simulink model "PC_drone_Simulation"  (R2014a)
settings: Solver=ode45  StartTime=0  StopTime=20  FixedStep=0.02  MaxStep=0.06  RelTol=1e-3
model workspace (MAT data in the model file):
  Sig = Simulink.Signal
  Sig.DataType = 'auto'
  Sig.Dimensions = -1
  Sig.DimensionsMode = 'auto'
  Sig.Complexity = 'auto'
  Sig.SampleTime = -1
  Sig.SamplingMode = 'auto'
Description:
  | This is a configurable quadcopter simulation.
  | This Simulink model demonstates attitude control.
  | 
  | Additional quadcopter modeling and simulation materials available at:
  | github.com/dch33/Quad-Sim
  | 
  | Copyright (C) 2014 D. Hartman, K. Landis, S. Moreno, J. Kim, M. Mehrer
  | 
  | License:
  |     This program is free software: you can redistribute it and/or modify
  |     it under the terms of the GNU LESSER GENERAL PUBLIC LICENSE as published by
  |     the Free Software Foundation, either version 3 of the License, or
  |     (at your option) any later version.
  | 
  |     This program is distributed in the hope that it will be useful,
  |     but WITHOUT ANY WARRANTY; without even the implied warranty of
  |     MERCHANTABILITY or FITNESS FOR A PARTICULAR PURPOSE.  See the
  |     GNU General Public License for more details.
  | 
  |     You should have received a copy of the GNU LESSER GENERAL PUBLIC LICENSE
  |     along with this program.  If not, see <http://www.gnu.org/licenses/>.
settings Model: ModifiedComment=USER -- Fri Dec 16 02:54:01 2016 -- Version 1.130  Creator=David Hartman  LastModifiedBy=khsun
settings Model: ModifiedHistory=|
  | USER -- Fri Dec 16 02:54:01 2016 -- Version 1.130
  | 
  | 
  | USER -- Fri Dec 16 02:54:01 2016 -- Version 1.130
  | 
  | 
  | USER -- Fri Dec 16 02:34:16 2016 -- Version 1.127
  | 
  | 
  | USER -- Fri Dec 16 02:34:16 2016 -- Version 1.127
  | 
  | 
  | USER -- Fri Dec 16 02:34:16 2016 -- Version 1.127
  | 
  | 
  | USER -- Fri Dec 16 01:26:53 2016 -- Version 1.126
  | 
  | 
  | USER -- Fri Dec 16 01:24:30 2016 -- Version 1.125
  | 
  | 
  | USER -- Fri Dec 16 01:23:22 2016 -- Version 1.124
  | 
  | 
  | USER -- Fri Dec 16 01:18:41 2016 -- Version 1.123
  | 
  | 
  | USER -- Fri Dec 16 01:06:27 2016 -- Version 1.121
  | 
  | 
  | USER -- Fri Dec 16 01:06:27 2016 -- Version 1.121
  | 
  | 
  | USER -- Fri Dec 16 01:06:15 2016 -- Version 1.120
  | 
  | 
  | USER -- Fri Dec 16 01:03:01 2016 -- Version 1.119
  | 
  | 
  | USER -- Fri Dec 16 01:02:34 2016 -- Version 1.118
  | 
  | 
  | USER -- Fri Dec 16 01:00:57 2016 -- Version 1.117
  | 
  | 
  | USER -- Fri Dec 16 00:59:40 2016 -- Version 1.116
  | 
  | 
  | USER -- Fri Dec 16 00:53:32 2016 -- Version 1.114
  | 
  | 
  | USER -- Fri Dec 16 00:53:32 2016 -- Version 1.114
  | 
  | 
  | USER -- Fri Dec 16 00:52:02 2016 -- Version 1.113
  | 
  | 
  | USER -- Fri Dec 16 00:41:04 2016 -- Version 1.112
  | 
  | 
  | USER -- Fri Dec 16 00:30:29 2016 -- Version 1.111
  | 
  | 
  | sstal -- Sun Dec 04 04:26:47 2016 -- Version 1.110
  | 
  | 
  | sstal -- Sun Dec 04 02:45:09 2016 -- Version 1.109
  | 
  | 
  | sstal -- Sun Dec 04 02:38:56 2016 -- Version 1.108
  | 
  | 
  | sstal -- Sun Dec 04 02:33:04 2016 -- Version 1.107
  | 
  | 
  | sstal -- Sun Dec 04 02:24:27 2016 -- Version 1.106
  | 
  | 
  | sstal -- Sun Dec 04 02:10:13 2016 -- Version 1.105
  | 
  | 
  | sstal -- Sun Dec 04 02:09:16 2016 -- Version 1.104
  | 
  | 
  | sstal -- Sun Dec 04 01:58:29 2016 -- Version 1.103
  | 
  | 
  | sstal -- Sun Dec 04 01:49:36 2016 -- Version 1.102
  | 
  | 
  | sstal -- Sat Dec 03 22:54:16 2016 -- Version 1.101
  | 
  | 
  | sstal -- Sat Dec 03 22:52:17 2016 -- Version 1.100
  | 
  | 
  | sstal -- Fri Dec 02 21:35:40 2016 -- Version 1.99
  | 
  | 
  | sstal -- Fri Dec 02 20:50:23 2016 -- Version 1.98
  | 
  | 
  | sstal -- Fri Dec 02 19:45:10 2016 -- Version 1.97
  | 
  | 
  | sstal -- Fri Dec 02 16:57:20 2016 -- Version 1.96
  | 
  | 
  | SKY 05 -- Fri Dec 02 00:32:51 2016 -- Version 1.95
  | 
  | 
  | SKY 05 -- Thu Dec 01 23:20:58 2016 -- Version 1.94
  | 
  | 
  | SKY 05 -- Thu Dec 01 12:57:28 2016 -- Version 1.93
  | 
  | 
  | SKY 05 -- Wed Nov 30 14:36:02 2016 -- Version 1.92
  | 
  | 
  | SKY 03 -- Tue Nov 29 23:04:25 2016 -- Version 1.91
  | 
  | 
  | SKY 03 -- Tue Nov 29 22:01:09 2016 -- Version 1.90
  | 
  | 
  | SKY 03 -- Tue Nov 29 21:15:44 2016 -- Version 1.89
  | 
  | 
  | SKY 03 -- Tue Nov 29 19:16:05 2016 -- Version 1.88
  | 
  | 
  | SKY 03 -- Tue Nov 29 18:05:54 2016 -- Version 1.87
  | 
  | 
  | SKY 03 -- Tue Nov 29 14:57:27 2016 -- Version 1.86
  | 
  | 
  | SKY 03 -- Tue Nov 29 14:50:24 2016 -- Version 1.85
  | 
  | 
  | SKY 03 -- Tue Nov 29 14:29:54 2016 -- Version 1.84
  | 
  | 
  | SKY 03 -- Tue Nov 29 14:29:26 2016 -- Version 1.83
  | 
  | 
  | SKY 03 -- Tue Nov 29 14:12:46 2016 -- Version 1.82
  | 
  | 
  | SKY 05 -- Tue Nov 29 01:43:26 2016 -- Version 1.81
  | 
  | 
  | SKY 05 -- Tue Nov 29 00:54:08 2016 -- Version 1.80
  | 
  | 
  | SKY 05 -- Tue Nov 29 00:24:35 2016 -- Version 1.79
  | 
  | 
  | SKY 05 -- Tue Nov 29 00:14:25 2016 -- Version 1.78
  | 
  | 
  | SKY 05 -- Tue Nov 29 00:11:46 2016 -- Version 1.77
  | 
  | 
  | SKY 05 -- Tue Nov 29 00:10:44 2016 -- Version 1.76
  | 
  | 
  | SKY 05 -- Mon Nov 28 23:29:36 2016 -- Version 1.75
  | 
  | 
  | SKY 05 -- Mon Nov 28 23:29:19 2016 -- Version 1.74
  | 
  | 
  | SKY 05 -- Mon Nov 28 23:23:54 2016 -- Version 1.73
  | 
  | 
  | SKY 05 -- Mon Nov 28 17:23:20 2016 -- Version 1.72
  | 
  | 
  | SKY 05 -- Mon Nov 28 15:05:10 2016 -- Version 1.71
  | 
  | 
  | SKY 05 -- Mon Nov 28 15:03:54 2016 -- Version 1.70
  | 
  | 
  | SKY 05 -- Mon Nov 28 15:01:18 2016 -- Version 1.69
  | 
  | 
  | SKY 05 -- Mon Nov 28 14:59:20 2016 -- Version 1.68
  | 
  | 
  | SKY15 -- Tue Dec 27 23:01:23 2016 -- Version 1.67
  | 
  | 
  | SKY 05 -- Sun Nov 27 00:40:54 2016 -- Version 1.66
  | 
  | 
  | SKY 05 -- Sun Nov 27 00:39:41 2016 -- Version 1.65
  | 
  | 
  | SKY 05 -- Sun Nov 27 00:35:40 2016 -- Version 1.64
  | 
  | 
  | SKY 05 -- Sun Nov 27 00:31:30 2016 -- Version 1.63
  | 
  | 
  | SKY 05 -- Sat Nov 26 23:45:19 2016 -- Version 1.62
  | 
  | 
  | SKY 05 -- Sat Nov 26 22:11:47 2016 -- Version 1.61
  | 
  | 
  | SKY 05 -- Sat Nov 26 22:06:18 2016 -- Version 1.60
  | 
  | 
  | SKY 05 -- Sat Nov 26 21:42:29 2016 -- Version 1.59
  | 
  | 
  | khsun -- Sat Nov 26 20:51:23 2016 -- Version 1.58
  | 
  | 
  | khsun -- Sat Nov 26 20:25:48 2016 -- Version 1.57
  | 
  | 
  | khsun -- Sat Nov 26 20:20:04 2016 -- Version 1.56
  | 
  | 
  | khsun -- Sat Nov 26 20:15:53 2016 -- Version 1.55
  | 
  | 
  | khsun -- Sat Nov 26 19:10:38 2016 -- Version 1.54
  | 
  | 
  | khsun -- Sat Nov 26 18:25:01 2016 -- Version 1.53
  | 
  | 
  | khsun -- Sat Nov 26 17:24:24 2016 -- Version 1.52
  | 
  | 
  | khsun -- Sat Nov 26 17:17:34 2016 -- Version 1.51
  | 
  | 
  | khsun -- Sat Nov 26 16:55:15 2016 -- Version 1.50
  | 
  | 
  | khsun -- Sat Nov 26 16:52:55 2016 -- Version 1.49
  | 
  | 
  | khsun -- Sat Nov 26 16:49:39 2016 -- Version 1.48
  | 
  | 
  | khsun -- Sat Nov 26 16:21:13 2016 -- Version 1.47
  | 
  | 
  | khsun -- Sat Nov 26 16:21:01 2016 -- Version 1.46
  | 
  | 
  | khsun -- Sat Nov 26 16:20:27 2016 -- Version 1.45
  | 
  | 
  | khsun -- Sat Nov 26 12:23:16 2016 -- Version 1.44
  | 
  | 
  | khsun -- Sat Nov 26 12:22:44 2016 -- Version 1.43
  | 
  | 
  | khsun -- Sat Nov 26 12:09:40 2016 -- Version 1.42
  | 
  | 
  | khsun -- Fri Nov 25 12:53:36 2016 -- Version 1.41
  | 
  | 
  | khsun -- Thu Nov 24 15:51:55 2016 -- Version 1.40
  | 
  | 
  | khsun -- Thu Nov 24 15:40:52 2016 -- Version 1.39
  | 
  | 
  | khsun -- Thu Nov 24 15:25:38 2016 -- Version 1.38
  | 
  | 
  | khsun -- Thu Nov 24 15:20:43 2016 -- Version 1.37
  | 
  | 
  | khsun -- Thu Nov 24 15:15:05 2016 -- Version 1.36
  | 
  | 
  | khsun -- Thu Nov 24 15:14:02 2016 -- Version 1.35
  | 
  | 
  | khsun -- Thu Nov 24 11:17:00 2016 -- Version 1.34
  | 
  | 
  | khsun -- Wed Nov 23 23:17:43 2016 -- Version 1.33
  | 
  | 
  | khsun -- Wed Nov 23 17:41:56 2016 -- Version 1.31
  | 
  | 
  | khsun -- Wed Nov 23 17:41:56 2016 -- Version 1.31
  | 
  | 
  | khsun -- Tue Nov 22 22:20:06 2016 -- Version 1.30
  | 
  | 
  | khsun -- Tue Nov 22 22:09:32 2016 -- Version 1.29
  | 
  | 
  | khsun -- Tue Nov 22 22:08:32 2016 -- Version 1.28
  | 
  | 
  | khsun -- Tue Nov 22 22:07:24 2016 -- Version 1.27
  | 
  | 
  | khsun -- Tue Nov 22 22:06:29 2016 -- Version 1.26
  | 
  | 
  | khsun -- Tue Nov 22 22:06:06 2016 -- Version 1.25
  | 
  | 
  | khsun -- Tue Nov 22 22:03:53 2016 -- Version 1.24
  | 
  | 
  | khsun -- Tue Nov 22 21:01:42 2016 -- Version 1.23
  | 
  | 
  | khsun -- Tue Nov 22 20:59:39 2016 -- Version 1.22
  | 
  | 
  | khsun -- Tue Nov 22 20:24:50 2016 -- Version 1.21
  | 
  | 
  | khsun -- Tue Nov 22 20:14:42 2016 -- Version 1.20
  | 
  | 
  | khsun -- Tue Nov 22 16:24:10 2016 -- Version 1.19
  | 
  | 
  | khsun -- Tue Nov 22 16:10:18 2016 -- Version 1.18
  | 
  | 
  | khsun -- Tue Nov 22 11:35:43 2016 -- Version 1.17
  | 
  | 
  | khsun -- Tue Nov 22 10:54:15 2016 -- Version 1.16
  | 
  | 
  | khsun -- Mon Nov 21 21:57:53 2016 -- Version 1.15
  | 
  | 
  | khsun -- Mon Nov 21 21:12:45 2016 -- Version 1.14
  | 
  | 
  | khsun -- Sun Nov 20 22:34:28 2016 -- Version 1.13
  | 
  | 
  | khsun -- Sun Nov 20 19:39:17 2016 -- Version 1.12
  | 
  | 
  | khsun -- Sun Nov 20 17:26:15 2016 -- Version 1.11
  | 
  | 
  | khsun -- Sun Nov 20 17:01:09 2016 -- Version 1.10
  | 
  | 
  | khsun -- Sun Nov 20 15:27:38 2016 -- Version 1.9
  | 
  | 
  | khsun -- Sun Nov 20 15:24:18 2016 -- Version 1.8
  | 
  | 
  | khsun -- Sun Nov 20 15:24:12 2016 -- Version 1.7
  | 
  | 
  | khsun -- Sun Nov 20 14:36:24 2016 -- Version 1.6
  | 
  | 
  | davidhartman -- Fri Jun 06 23:19:51 2014 -- Version 1.5
  | 
  | 
  | davidhartman -- Fri Jun 06 22:53:10 2014 -- Version 1.3
settings SolverCC: AutoInsertRateTranBlk=on
settings DataIOCC: LimitDataPoints=off  SignalLogging=off
settings OptimizationCC: InlineParams=on
settings DebuggingCC: UnderspecifiedInitializationDetection=Classic  UniqueDataStoreMsg=warning  StateNameClashWarn=warning  StrictBusMsg=WarnOnBusTreatedAsVector

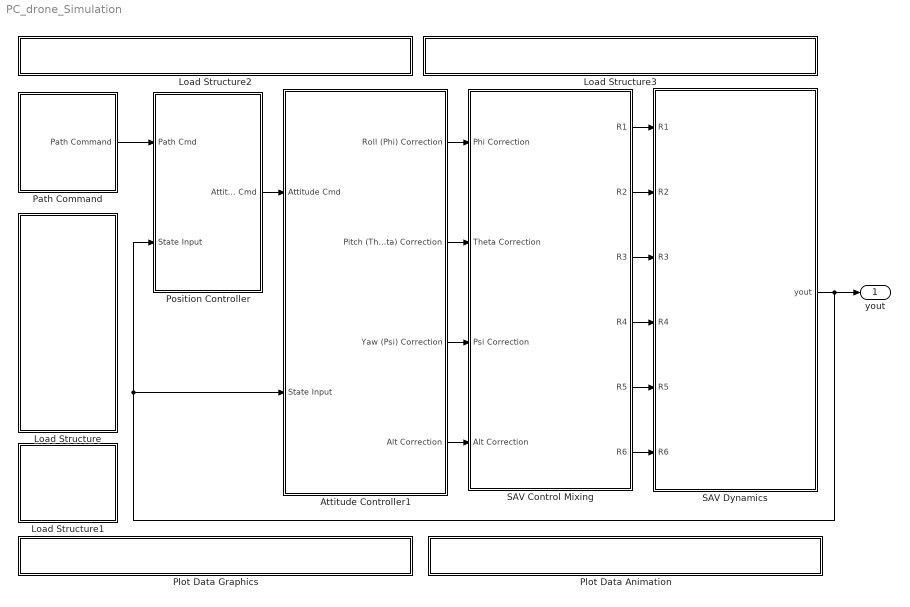
== system PC_drone_Simulation ==
  Attitude Controller1 : Subsystem
  Load Structure : Subsystem
      settings: OpenFcn=|
      | uiopen('load')
      | if ((exist('IC')==1) && (exist('quadModel')==1) && (exist('path')==1))
      | set_param(bdroot, 'SimulationCommand', 'update')
      | end
      mask Display: fprintf('LOAD:\nTimeseries\nPath\nCommands,\ndrone\nModel, Or\nInitial\nConditions');
  Load Structure1 : Subsystem
      settings: OpenFcn=|
      | if (exist('IC')==1 && exist('quadModel')==1 && exist('yout') && exist('tout'))
      | saveSimResults()
      | else
      | msgbox('No Data To Save!')
      | end
      mask Display: fprintf('SAVE:\nSimulation\nResults');
  Load Structure2 : Subsystem
      settings: OpenFcn=|
      | if exist('GUI_Modeling') == 2,
      | run('GUI_Modeling')
      | 
      | else
      | 
      | msgbox('The desired GUI must be first added to MATLABs path.')
      | 
      | end
      mask Display: fprintf('OPEN GUI: Build New \n Model');
  Load Structure3 : Subsystem
      settings: OpenFcn=|
      | if exist('GUI_IC') == 2,
      | run('GUI_IC')
      | 
      | else
      | 
      | msgbox('The desired GUI must be first added to MATLABs path.')
      | 
      | end
      mask Display: fprintf('OPEN GUI: Create Initial \n Conditions');
  Path Command : Subsystem  mask{Interpolate=on, OutputAfterFinalValue=Holding final value}
      mask prompts: Interpolate "Interpolate X, Y, Z, and Psi command data?"; OutputAfterFinalValue "Form output after final data value by:"
      mask help:
      | Selecting the Interpolate data checkbox causes position commands to be
      | linearly interpolated. For additional options related to the Timeseries
      | "path" commands, look under the block and click on the Timeseries From
      | Workspace blocks.
      mask TypeOptions Interpolate: X Timeseries From Wkspace/Interpolate | Y Timeseries From Wkspace/Interpolate | Z Timeseries From Wkspace/Interpolate | Psi Timeseries From Wkspace/Interpolate
      mask TypeOptions OutputAfterFinalValue: X Timeseries From Wkspace/OutputAfterFinalValue | Y Timeseries From Wkspace/OutputAfterFinalValue | Z Timeseries From Wkspace/OutputAfterFinalValue | Psi Timeseries From Wkspace/OutputAfterFinalValue
  Plot Data Animation : Subsystem
      settings: OpenFcn=|
      | if exist('droneAnim4') == 2,
      |     if exist('yout')
      | 	run('droneAnim4');
      |     else
      |     msgbox('Simulation must be run before data can be plotted.');
      |     end
      | else                                                                          msgbox('The desired GUI must be first added to MATLABs path.')
      | end
      mask Display: fprintf('OPEN GUI: Flight Animation')
  Plot Data Graphics : Subsystem
      settings: OpenFcn=|
      | if exist('yout')
      | yout = evalin('base', 'yout');
      | tout = evalin('base', 'tout');
      | dronePlots(yout, tout)
      | else
      | msgbox('Simulation must be run before data can be plotted.')
      | end
      mask Display: fprintf('OPEN PLOT: State Data')
  Position Controller : Subsystem
  SAV Control Mixing : Subsystem
  SAV Dynamics : Subsystem
  yout : Outport
  wires:
  Position Controller/1(Attitude Cmd) -> Attitude Controller1/1(Attitude Cmd)
  Path Command/1("Path Command ") -> Position Controller/1(Path Cmd)
  Attitude Controller1/1(Roll (Phi) Correction) -> SAV Control Mixing/1(Phi Correction)
  Attitude Controller1/2(Pitch (Theta) Correction) -> SAV Control Mixing/2(Theta Correction)
  Attitude Controller1/3(Yaw (Psi) Correction) -> SAV Control Mixing/3(Psi Correction)
  Attitude Controller1/4(Alt Correction) -> SAV Control Mixing/4(Alt Correction)
  SAV Control Mixing/1(R1) -> SAV Dynamics/1(R1)
  SAV Control Mixing/2(R2) -> SAV Dynamics/2(R2)
  SAV Control Mixing/3(R3) -> SAV Dynamics/3(R3)
  SAV Control Mixing/4(R4) -> SAV Dynamics/4(R4)
  SAV Control Mixing/5(R5) -> SAV Dynamics/5(R5)
  SAV Control Mixing/6(R6) -> SAV Dynamics/6(R6)
  SAV Dynamics/1(yout) -> Attitude Controller1/2(State Input), Position Controller/2(State Input), yout/1

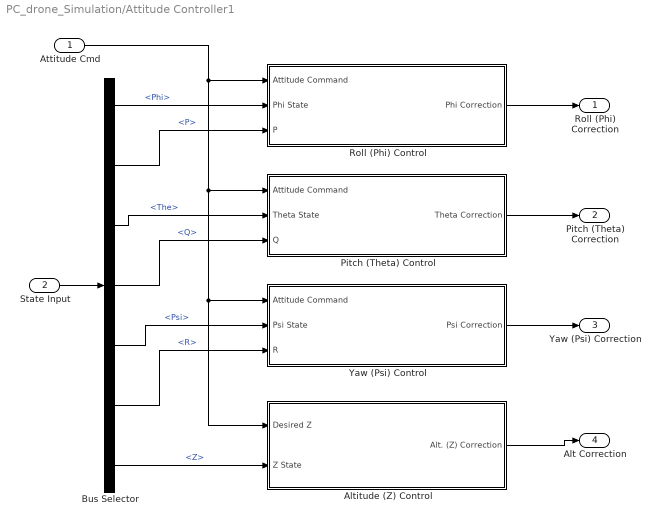
== system PC_drone_Simulation/Attitude Controller1 ==
  Attitude Cmd : Inport
  State Input : Inport  Port=2
  Altitude (Z) Control : Subsystem  mask{Kpz=10, Kiz=0, Kdz=3, LimitOutput=off, USat=1, LSat=-1, GOffset=0}
      mask prompts: Kpz "Kp"; Kiz "Ki"; Kdz "Kd"; LimitOutput "Integral Saturation?"; USat "Upper saturation limit:"; LSat "Lower saturation limit:"; GOffset "Gravity Feedforward"
      mask help:
      | Adjust PID controller gains through this mask interface, or "look under mask" for more detailed adjustments.
      |
      | Note: Gravity Offset will not appear on block face as a value until simulation is run if it is the result of a formula involving the quadcopter model parameters.
      mask TypeOptions Kpz: Kpz/Gain
      mask TypeOptions Kiz: Kiz/Gain
      mask TypeOptions Kdz: Kdz/Gain
      mask TypeOptions LimitOutput:
      | Integrator
      | Limited/LimitOutput
      mask TypeOptions USat:
      | Integrator
      | Limited/UpperSaturationLimit
      mask TypeOptions LSat:
      | Integrator
      | Limited/LowerSaturationLimit
      mask TypeOptions GOffset: Gravity Offset (Level Flight)/Value
      mask Display:
      | fprintf(['Kp = ' num2str(Kpz) '\n' ...
      |     'Ki = ' num2str(Kiz) '\n' ...
      |     'Kd = ' num2str(Kdz) '\n' ...
      |     'Integral Saturation: ' LimitOutput]);
      | if strcmp(LimitOutput,'on')
      |     fprintf([' \n' ' \n' ' \n' ' \n' ' \n' '\n' ...
      |         'Limits: ' num2str(USat) ' to ' num2str(LSat)]);
      | end
  Bus Selector : BusSelector  OutputSignals=Phi,P,The,Q,Psi,R,Z
  Pitch (Theta) Control : Subsystem  mask{Kpt=5, Kit=1, Kdt=3, LimitOutput=off, USat=1, LSat=-1}
      mask prompts: Kpt "Kp"; Kit "Ki"; Kdt "Kd"; LimitOutput "Integral Saturation?"; USat "Upper saturation limit:"; LSat "Lower saturation limit:"
      mask help: Adjust PID controller gains through this mask interface, or "look under mask" for more detailed adjustments.
      mask TypeOptions Kpt: Kpt/Gain
      mask TypeOptions Kit: Kit/Gain
      mask TypeOptions Kdt: Kdt/Gain
      mask TypeOptions LimitOutput:
      | Integrator
      | Limited/LimitOutput
      mask TypeOptions USat:
      | Integrator
      | Limited/UpperSaturationLimit
      mask TypeOptions LSat:
      | Integrator
      | Limited/LowerSaturationLimit
      mask Display:
      | fprintf(['Kp = ' num2str(Kpt) '\n' ...
      |     'Ki = ' num2str(Kit) '\n' ...
      |     'Kd = ' num2str(Kdt) '\n' ...
      |     'Integral Saturation: ' LimitOutput]);
      | if strcmp(LimitOutput,'on')
      |     fprintf([' \n' ' \n' ' \n' ' \n' '\n' ...
      |         'Limits: ' num2str(USat) ' to ' num2str(LSat)]);
      | end
  "Roll (Phi) Control " : Subsystem  mask{Kpp=5, Kip=1, Kdp=3, LimitOutput=off, USat=1, LSat=-1}
      mask prompts: Kpp "Kp"; Kip "Ki"; Kdp "Kd"; LimitOutput "Integral Saturation:"; USat "Upper saturation limit:"; LSat "Lower saturation limit:"
      mask help:
      | Adjust PID controller gains through this mask interface, or "look under mask"
      | for more detailed adjustments.
      mask TypeOptions Kpp: Kpp/Gain
      mask TypeOptions Kip: Kip/Gain
      mask TypeOptions Kdp: Kdp/Gain
      mask TypeOptions LimitOutput:
      | Integrator
      | Limited/LimitOutput
      mask TypeOptions USat:
      | Integrator
      | Limited/UpperSaturationLimit
      mask TypeOptions LSat:
      | Integrator
      | Limited/LowerSaturationLimit
      mask Display:
      | fprintf(['Kp = ' num2str(Kpp) '\n' ...
      |     'Ki = ' num2str(Kip) '\n' ...
      |     'Kd = ' num2str(Kdp) '\n'...
      |     'Integral Saturation: ' LimitOutput]);
      | if strcmp(LimitOutput,'on')
      |     fprintf([' \n' ' \n' ' \n' ' \n' '\n' ...
      |         'Limits: ' num2str(USat) ' to ' num2str(LSat)]);
      | end
  Yaw (Psi) Control : Subsystem  mask{Kps=4, Kis=1, Kds=2, LimitOutput=off, USat=1, LSat=-1}
      mask prompts: Kps "Kp"; Kis "Ki"; Kds "Kd"; LimitOutput "Integral Saturation?"; USat "Upper saturation limit:"; LSat "Lower saturation limit:"
      mask help: Adjust PID controller gains through this mask interface, or "look under mask" for more detailed adjustments.
      mask TypeOptions Kps: Kps/Gain
      mask TypeOptions Kis: Kit/Gain
      mask TypeOptions Kds: Kds/Gain
      mask TypeOptions LimitOutput:
      | Integrator
      | Limited/LimitOutput
      mask TypeOptions USat:
      | Integrator
      | Limited/UpperSaturationLimit
      mask TypeOptions LSat:
      | Integrator
      | Limited/LowerSaturationLimit
      mask Display:
      | fprintf(['Kp = ' num2str(Kps) '\n' ...
      |     'Ki = ' num2str(Kis) '\n' ...
      |     'Kd = ' num2str(Kds) '\n' ...
      |     'Integral Saturation: ' LimitOutput]);
      | if strcmp(LimitOutput,'on')
      |     fprintf([' \n' ' \n' ' \n' ' \n' '\n' ...
      |         'Limits: ' num2str(USat) ' to ' num2str(LSat)]);
      | end
  Roll (Phi) Correction : Outport
  Pitch (Theta) Correction : Outport  Port=2
  Yaw (Psi) Correction : Outport  Port=3
  Alt Correction : Outport  Port=4
  wires:
  Bus Selector/3 -> Pitch (Theta) Control/2(Theta State)  "<The>"
  Attitude Cmd/1 -> Altitude (Z) Control/1(Desired Z), Yaw (Psi) Control/1(Attitude Command), Pitch (Theta) Control/1(Attitude Command), "Roll (Phi) Control "/1("Attitude Command ")
  Bus Selector/5 -> Yaw (Psi) Control/2(Psi State)  "<Psi>"
  Yaw (Psi) Control/1(Psi Correction) -> Yaw (Psi) Correction/1
  Pitch (Theta) Control/1(Theta Correction) -> Pitch (Theta) Correction/1
  State Input/1 -> Bus Selector/1
  Bus Selector/1 -> "Roll (Phi) Control "/2(Phi State)  "<Phi>"
  "Roll (Phi) Control "/1(Phi Correction) -> Roll (Phi) Correction/1
  Bus Selector/7 -> Altitude (Z) Control/2(Z State)  "<Z>"
  Altitude (Z) Control/1(Alt. (Z) Correction) -> Alt Correction/1
  Bus Selector/2 -> "Roll (Phi) Control "/3(P)  "<P>"
  Bus Selector/4 -> Pitch (Theta) Control/3(Q)  "<Q>"
  Bus Selector/6 -> Yaw (Psi) Control/3(R)  "<R>"

== system PC_drone_Simulation/Load Structure ==

== system PC_drone_Simulation/Load Structure1 ==

== system PC_drone_Simulation/Load Structure2 ==

== system PC_drone_Simulation/Load Structure3 ==

== system PC_drone_Simulation/Path Command ==
  Bus Creator : BusCreator  Inputs=3
  Bus Selector : BusSelector  OutputSignals=X_cmd,Y_cmd  OutputAsBus=on
  X Timeseries From Wkspace : FromWorkspace  VariableName=path.x  SampleTime=0  OutputAfterFinalValue=Holding final value
  Y Timeseries From Wkspace : FromWorkspace  VariableName=path.y  SampleTime=0  OutputAfterFinalValue=Holding final value
  Z Timeseries From Wkspace : FromWorkspace  VariableName=path.z  SampleTime=0  OutputAfterFinalValue=Holding final value
  "Path Command " : Outport
  tag scope: C=global
  wires:
  X Timeseries From Wkspace/1 -> Bus Creator/1  "X_cmd"
  Y Timeseries From Wkspace/1 -> Bus Creator/2  "Y_cmd"
  Z Timeseries From Wkspace/1 -> Bus Creator/3  "Alt_Cmd"
  Bus Creator/1 -> "Path Command "/1, Bus Selector/1  "Path_Cmd"
  Bus Selector/1 -> [C]  "XY_Cmd"

== system PC_drone_Simulation/Plot Data Animation ==

== system PC_drone_Simulation/Plot Data Graphics ==

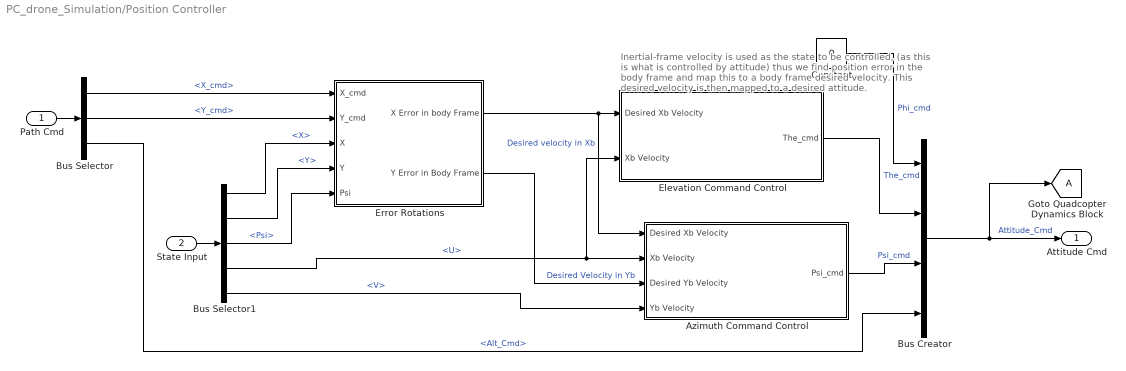
== system PC_drone_Simulation/Position Controller ==
  note: Inertial-frame velocity is used as the state to be controlled,
      | (as this is what is controlled by attitude)
      | thus we find position error in the body frame
      | and map this to a body frame desired velocity. This desired
      | velocity is then mapped to a desired attitude.
  Path Cmd : Inport
  State Input : Inport  Port=2
  Azimuth Command Control : Subsystem  mask{Kp=0.3, Kd=0}
      mask prompts: Kp "Proportional Gain"; Kd "Derivative Gain"
      mask TypeOptions Kp: Kpp/Gain
      mask TypeOptions Kd: Kdp/Gain
      mask Display:
      | fprintf(['Kp = ' num2str(Kp) '\n' ...
      |     'Kd = ' num2str(Kd) '\n']);
  Bus Creator : BusCreator  Inputs='Phi_cmd','The_cmd','Psi_cmd','Alt_Cmd'
  Bus Selector : BusSelector  OutputSignals=X_cmd,Y_cmd,Alt_Cmd
  Bus Selector1 : BusSelector  OutputSignals=X,Y,Psi,U,V
  Constant : Constant  Value=0
  Elevation Command Control : Subsystem  mask{Kp=0.3, Kd=0, ASat=30*pi/180}
      mask prompts: Kp "Proportional Gain:"; Kd "Derivative Gain"; ASat "Attitude Limit (+/- radians):"
      mask TypeOptions Kp: Kpt/Gain
      mask TypeOptions Kd: Kdt/Gain
      mask TypeOptions ASat: Attitude Limits_Theta/UpperLimit
      mask Display:
      | fprintf(['Kp = ' num2str(Kp) '\n' ...
      |     'Kd = ' num2str(Kd) '\n' ...
      |     'Attitude Limit (+/-): ' num2str(ASat*180/pi) '°']);
  Error Rotations : Subsystem
  Attitude Cmd : Outport
  tag scope: A=global
  wires:
  State Input/1 -> Bus Selector1/1
  Path Cmd/1 -> Bus Selector/1
  Bus Creator/1 -> [A], Attitude Cmd/1  "Attitude_Cmd"
  Bus Selector/1 -> Error Rotations/1(X_cmd)  "<X_cmd>"
  Bus Selector/2 -> Error Rotations/2(Y_cmd)  "<Y_cmd>"
  Bus Selector1/1 -> Error Rotations/3(X)  "<X>"
  Bus Selector1/2 -> Error Rotations/4(Y)  "<Y>"
  Bus Selector1/3 -> Error Rotations/5(Psi)  "<Psi>"
  Constant/1 -> Bus Creator/1  "Phi_cmd"
  Elevation Command Control/1(The_cmd) -> Bus Creator/2  "The_cmd"
  Error Rotations/1(X Error in body Frame) -> Azimuth Command Control/1(Desired Xb Velocity), Elevation Command Control/1(Desired Xb Velocity)  "Desired velocity in Xb"
  Error Rotations/2(Y Error in Body Frame) -> Azimuth Command Control/3(Desired Yb Velocity)  "Desired Velocity in Yb"
  Bus Selector1/4 -> Elevation Command Control/2(Xb Velocity), Azimuth Command Control/2(Xb Velocity)  "<U>"
  Bus Selector1/5 -> Azimuth Command Control/4(Yb Velocity)  "<V>"
  Bus Selector/3 -> Bus Creator/4  "<Alt_Cmd>"
  Azimuth Command Control/1(Psi_cmd) -> Bus Creator/3  "Psi_cmd"

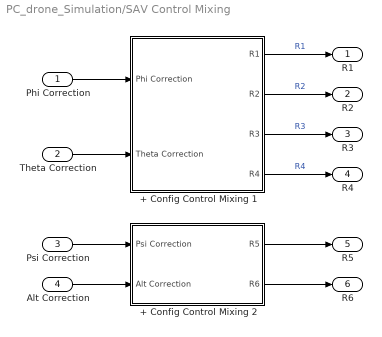
== system PC_drone_Simulation/SAV Control Mixing ==
  Phi Correction : Inport
  Theta Correction : Inport  Port=2
  Psi Correction : Inport  Port=3
  Alt Correction : Inport  Port=4
  + Config Control Mixing 1 : Subsystem
  + Config Control Mixing 2 : Subsystem
  R1 : Outport
  R2 : Outport  Port=2
  R3 : Outport  Port=3
  R4 : Outport  Port=4
  R5 : Outport  Port=5
  R6 : Outport  Port=6
  wires:
  + Config Control Mixing 1/4(R4) -> R4/1  "R4"
  + Config Control Mixing 1/3(R3) -> R3/1  "R3"
  + Config Control Mixing 1/2(R2) -> R2/1  "R2"
  + Config Control Mixing 1/1(R1) -> R1/1  "R1"
  Theta Correction/1 -> + Config Control Mixing 1/2(Theta Correction)
  Phi Correction/1 -> + Config Control Mixing 1/1(Phi Correction)
  Psi Correction/1 -> + Config Control Mixing 2/1(Psi Correction)
  Alt Correction/1 -> + Config Control Mixing 2/2(Alt Correction)
  + Config Control Mixing 2/1(R5) -> R5/1
  + Config Control Mixing 2/2(R6) -> R6/1

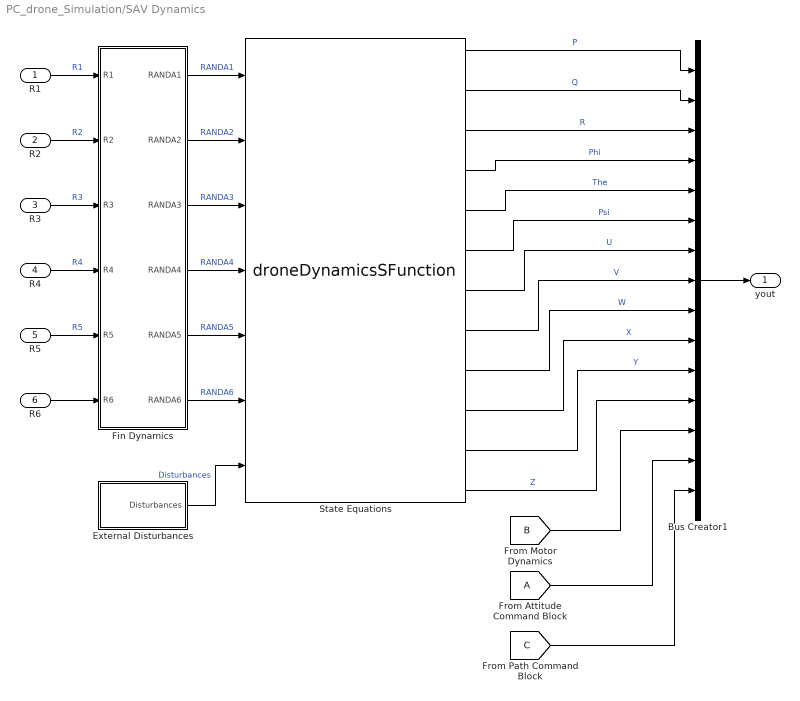
== system PC_drone_Simulation/SAV Dynamics ==
  R1 : Inport
  R2 : Inport  Port=2
  R3 : Inport  Port=3
  R4 : Inport  Port=4
  R5 : Inport  Port=5
  R6 : Inport  Port=6
  Bus Creator1 : BusCreator  Inputs='P','Q','R','Phi','The','Psi','U','V','W','X','Y','Z','mc and RPM','Attitude_Cmd','XY_Cmd'
  External Disturbances : Subsystem
  Fin Dynamics : Subsystem  mask{AOA=50*pi/180}
      mask prompts: AOA "Simulink:blkprm_prompts:SaturateUpLim"
      mask TypeOptions AOA: Signal_Saturation_1/UpperLimit | Signal_Saturation_2/UpperLimit | Signal_Saturation_3/UpperLimit | Signal_Saturation_4/UpperLimit
      mask Display: fprintf(['AOA = ' num2str(AOA*180/pi) '°']);
  State Equations : M-S-Function  FunctionName=droneDynamicsSFunction  Parameters=droneModel, IC
      mask Display:
      | port_label('input', 1, 'RANDA1')
      | port_label('input', 2, 'RANDA2')
      | port_label('input', 3, 'RANDA3')
      | port_label('input', 4, 'RANDA4')
      | port_label('input', 5, 'RANDA5')
      | port_label('input', 6, 'RANDA6')
      | port_label('input', 7, 'Disturbances')
      | port_label('output', 1, 'P')
      | port_label('output', 2, 'Q')
      | port_label('output', 3, 'R')
      | port_label('output', 4, 'Phi')
      | port_label('output', 5, 'The')
      | port_label('output', 6, 'Psi')
      | port_label('output', 7, 'U')
      | port_label('output', 8, 'V')
      | port_label('output', 9, 'W')
      | port_label('output', 10, 'X')
      | port_label('output', 11, 'Y')
      | port_label('output', 12, 'Z')
  yout : Outport
  wires:
  [B] -> Bus Creator1/13
  [A] -> Bus Creator1/14
  R2/1 -> Fin Dynamics/2(R2)  "R2"
  R3/1 -> Fin Dynamics/3(R3)  "R3"
  R4/1 -> Fin Dynamics/4(R4)  "R4"
  R1/1 -> Fin Dynamics/1(R1)  "R1"
  Fin Dynamics/4(RANDA4) -> State Equations/4  "RANDA4"
  Fin Dynamics/3(RANDA3) -> State Equations/3  "RANDA3"
  Fin Dynamics/2(RANDA2) -> State Equations/2  "RANDA2"
  Fin Dynamics/1(RANDA1) -> State Equations/1  "RANDA1"
  State Equations/6 -> Bus Creator1/6  "Psi"
  State Equations/5 -> Bus Creator1/5  "The"
  State Equations/4 -> Bus Creator1/4  "Phi"
  State Equations/3 -> Bus Creator1/3  "R"
  State Equations/2 -> Bus Creator1/2  "Q"
  State Equations/1 -> Bus Creator1/1  "P"
  Bus Creator1/1 -> yout/1
  State Equations/12 -> Bus Creator1/12  "Z"
  State Equations/11 -> Bus Creator1/11  "Y"
  State Equations/10 -> Bus Creator1/10  "X"
  State Equations/9 -> Bus Creator1/9  "W"
  State Equations/7 -> Bus Creator1/7  "U"
  State Equations/8 -> Bus Creator1/8  "V"
  R5/1 -> Fin Dynamics/5(R5)  "R5"
  R6/1 -> Fin Dynamics/6(R6)
  Fin Dynamics/5(RANDA5) -> State Equations/5  "RANDA5"
  Fin Dynamics/6(RANDA6) -> State Equations/6  "RANDA6"
  External Disturbances/1("Disturbances ") -> State Equations/7  "Disturbances"
  [C] -> Bus Creator1/15

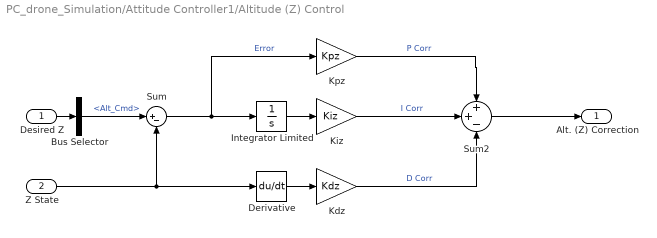
== system PC_drone_Simulation/Attitude Controller1/Altitude (Z) Control ==
  Desired Z : Inport
  Z State : Inport  Port=2
  Bus Selector : BusSelector  OutputSignals=Alt_Cmd
  Derivative : Derivative
  Integrator Limited : Integrator  UpperSaturationLimit=USat  LowerSaturationLimit=LSat
  Kdz : Gain  Gain=Kdz
  Kiz : Gain  Gain=Kiz
  Kpz : Gain  Gain=Kpz
  Sum : Sum  Inputs=|+-
  Sum2 : Sum  Inputs=++-
  Alt. (Z) Correction : Outport
  wires:
  Derivative/1 -> Kdz/1
  Bus Selector/1 -> Sum/1  "<Alt_Cmd>"
  Integrator Limited/1 -> Kiz/1
  Kdz/1 -> Sum2/3  "D Corr"
  Kpz/1 -> Sum2/1  "P Corr"
  Z State/1 -> Sum/2, Derivative/1
  Desired Z/1 -> Bus Selector/1
  Kiz/1 -> Sum2/2  "I Corr"
  Sum/1 -> Integrator Limited/1, Kpz/1  "Error"
  Sum2/1 -> Alt. (Z) Correction/1

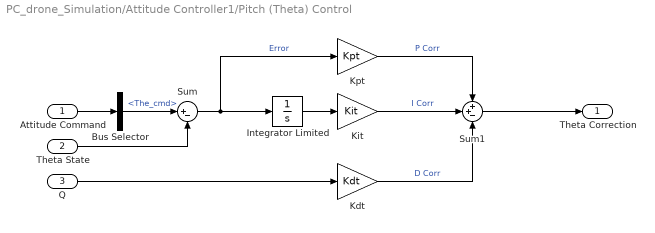
== system PC_drone_Simulation/Attitude Controller1/Pitch (Theta) Control ==
  Attitude Command : Inport
  Theta State : Inport  Port=2
  Q : Inport  Port=3
  Bus Selector : BusSelector  OutputSignals=The_cmd
  Integrator Limited : Integrator  UpperSaturationLimit=USat  LowerSaturationLimit=LSat
  Kdt : Gain  Gain=Kdt
  Kit : Gain  Gain=Kit
  Kpt : Gain  Gain=Kpt
  Sum : Sum  Inputs=|+-
  Sum1 : Sum  Inputs=++-
  Theta Correction : Outport
  wires:
  Bus Selector/1 -> Sum/1  "<The_cmd>"
  Integrator Limited/1 -> Kit/1
  Kit/1 -> Sum1/2  "I Corr"
  Kdt/1 -> Sum1/3  "D Corr"
  Kpt/1 -> Sum1/1  "P Corr"
  Sum1/1 -> Theta Correction/1
  Attitude Command/1 -> Bus Selector/1
  Sum/1 -> Kpt/1, Integrator Limited/1  "Error"
  Theta State/1 -> Sum/2
  Q/1 -> Kdt/1

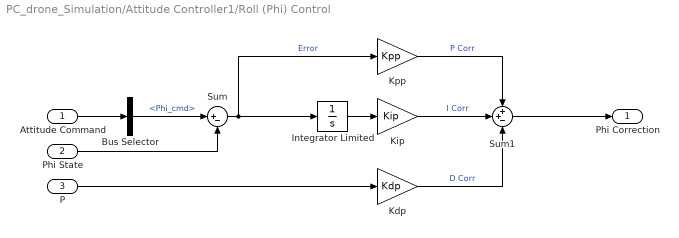
== system PC_drone_Simulation/Attitude Controller1/Roll (Phi) Control  ==
  "Attitude Command " : Inport
  Phi State : Inport  Port=2
  P : Inport  Port=3
  Bus Selector : BusSelector  OutputSignals=Phi_cmd
  Integrator Limited : Integrator  UpperSaturationLimit=USat  LowerSaturationLimit=LSat
  Kdp : Gain  Gain=Kdp
  Kip : Gain  Gain=Kip
  Kpp : Gain  Gain=Kpp
  Sum : Sum  Inputs=|+-
  Sum1 : Sum  Inputs=++-
  Phi Correction : Outport
  wires:
  Bus Selector/1 -> Sum/1  "<Phi_cmd>"
  "Attitude Command "/1 -> Bus Selector/1
  Integrator Limited/1 -> Kip/1
  Kip/1 -> Sum1/2  "I Corr"
  Kdp/1 -> Sum1/3  "D Corr"
  Kpp/1 -> Sum1/1  "P Corr"
  Sum1/1 -> Phi Correction/1
  Sum/1 -> Kpp/1, Integrator Limited/1  "Error"
  Phi State/1 -> Sum/2
  P/1 -> Kdp/1

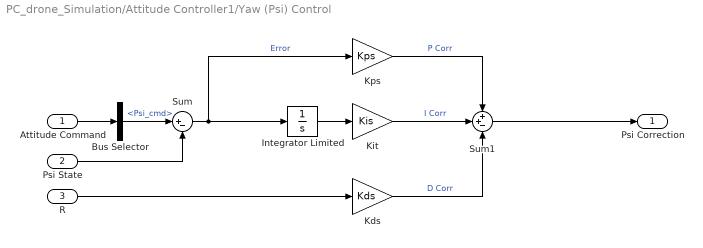
== system PC_drone_Simulation/Attitude Controller1/Yaw (Psi) Control ==
  Attitude Command : Inport
  Psi State : Inport  Port=2
  R : Inport  Port=3
  Bus Selector : BusSelector  OutputSignals=Psi_cmd
  Integrator Limited : Integrator  UpperSaturationLimit=USat  LowerSaturationLimit=LSat
  Kds : Gain  Gain=Kds
  Kit : Gain  Gain=Kis
  Kps : Gain  Gain=Kps
  Sum : Sum  Inputs=|+-
  Sum1 : Sum  Inputs=++-
  Psi Correction : Outport
  wires:
  Bus Selector/1 -> Sum/1  "<Psi_cmd>"
  Integrator Limited/1 -> Kit/1
  Kit/1 -> Sum1/2  "I Corr"
  Kds/1 -> Sum1/3  "D Corr"
  Kps/1 -> Sum1/1  "P Corr"
  Sum1/1 -> Psi Correction/1
  Attitude Command/1 -> Bus Selector/1
  Sum/1 -> Kps/1, Integrator Limited/1  "Error"
  R/1 -> Kds/1
  Psi State/1 -> Sum/2

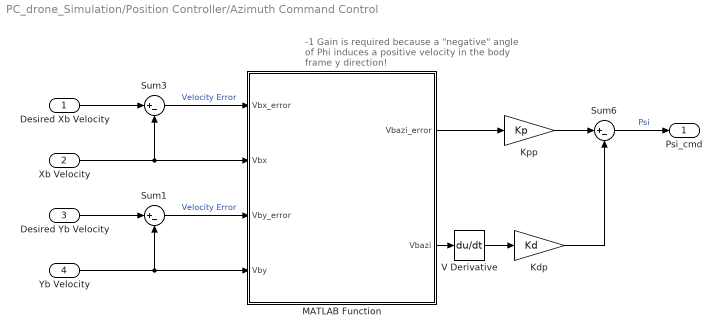
== system PC_drone_Simulation/Position Controller/Azimuth Command Control ==
  note: -1 Gain is required because a "negative"
      | angle of Phi induces a positive velocity
      | in the body frame y direction!
  Desired Xb Velocity : Inport
  Xb Velocity : Inport  Port=2
  Desired Yb Velocity : Inport  Port=3
  Yb Velocity : Inport  Port=4
  Kdp : Gain  Gain=Kd
  Kpp : Gain  Gain=Kp
  MATLAB Function : MATLAB Function  TreatAsAtomicUnit=on
  Sum1 : Sum  Inputs=|+-
  Sum3 : Sum  Inputs=|+-
  Sum6 : Sum  Inputs=|+-
  V Derivative : Derivative
  Psi_cmd : Outport
  wires:
  V Derivative/1 -> Kdp/1
  Kpp/1 -> Sum6/1
  Xb Velocity/1 -> Sum3/2, MATLAB Function/2(Vbx)
  Desired Xb Velocity/1 -> Sum3/1
  Kdp/1 -> Sum6/2
  Yb Velocity/1 -> Sum1/2, MATLAB Function/4(Vby)
  Desired Yb Velocity/1 -> Sum1/1
  Sum3/1 -> MATLAB Function/1(Vbx_error)  "Velocity Error"
  Sum1/1 -> MATLAB Function/3(Vby_error)  "Velocity Error"
  MATLAB Function/1(Vbazi_error) -> Kpp/1
  MATLAB Function/2(Vbazi) -> V Derivative/1
  Sum6/1 -> Psi_cmd/1  "Psi"

== system PC_drone_Simulation/Position Controller/Elevation Command Control ==
  Desired Xb Velocity : Inport
  Xb Velocity : Inport  Port=2
  Attitude Limits_Theta : Saturate  UpperLimit=ASat  LowerLimit=-ASat
  Kdt : Gain  Gain=Kd
  Kpt : Gain  Gain=Kp
  Sum3 : Sum  Inputs=|+-
  Sum6 : Sum  Inputs=|+-
  U Derivative : Derivative
  The_cmd : Outport
  wires:
  Kdt/1 -> Sum6/2
  U Derivative/1 -> Kdt/1
  Attitude Limits_Theta/1 -> The_cmd/1  "The_cmd"
  Sum6/1 -> Attitude Limits_Theta/1
  Kpt/1 -> Sum6/1
  Sum3/1 -> Kpt/1  "Velocity Error"
  Xb Velocity/1 -> U Derivative/1, Sum3/2
  Desired Xb Velocity/1 -> Sum3/1

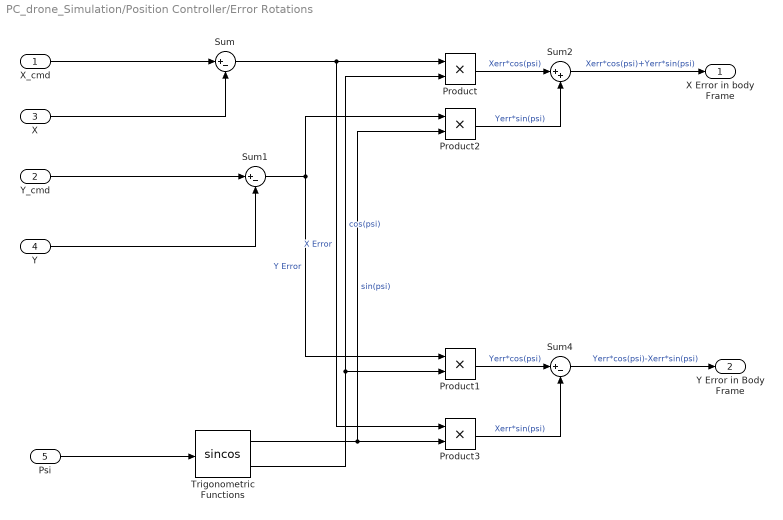
== system PC_drone_Simulation/Position Controller/Error Rotations ==
  X_cmd : Inport
  Y_cmd : Inport  Port=2
  X : Inport  Port=3
  Y : Inport  Port=4
  Psi : Inport  Port=5
  Product{,1..3} (4 alike) : Product
  Sum : Sum  Inputs=|+-
  Sum1 : Sum  Inputs=|+-
  Sum2 : Sum  Inputs=|++
  Sum4 : Sum  Inputs=|+-
  Trigonometric Functions : Trigonometry  Operator=sincos
  X Error in body Frame : Outport
  Y Error in Body Frame : Outport  Port=2
  wires:
  Sum4/1 -> Y Error in Body Frame/1  "Yerr*cos(psi)-Xerr*sin(psi)"
  Product3/1 -> Sum4/2  "Xerr*sin(psi)"
  Sum1/1 -> Product2/1, Product1/1  "Y Error"
  Trigonometric Functions/1 -> Product2/2, Product3/2  "sin(psi)"
  Sum2/1 -> X Error in body Frame/1  "Xerr*cos(psi)+Yerr*sin(psi)"
  Y_cmd/1 -> Sum1/1
  X_cmd/1 -> Sum/1
  X/1 -> Sum/2
  Y/1 -> Sum1/2
  Sum/1 -> Product3/1, Product/1  "X Error"
  Trigonometric Functions/2 -> Product/2, Product1/2  "cos(psi)"
  Product/1 -> Sum2/1  "Xerr*cos(psi)"
  Product2/1 -> Sum2/2  "Yerr*sin(psi)"
  Product1/1 -> Sum4/1  "Yerr*cos(psi)"
  Psi/1 -> Trigonometric Functions/1

== system PC_drone_Simulation/SAV Control Mixing/+ Config Control Mixing 1 ==
  note: mc1 = - The_cor
  note: mc3 = - The_cor
  note: mc4 = - Phi_cor
  note: + (plus) Drone Configuration Control Mixing
  note: mc2 = - Phi_cor
  Phi Correction : Inport
  Theta Correction : Inport  Port=2
  Sum{1..4} (4 alike) : Sum  Inputs=-
  R1 : Outport
  R2 : Outport  Port=2
  R3 : Outport  Port=3
  R4 : Outport  Port=4
  wires:
  Sum3/1 -> R3/1
  Sum1/1 -> R1/1
  Theta Correction/1 -> Sum1/1, Sum3/1
  Phi Correction/1 -> Sum4/1, Sum2/1
  Sum2/1 -> R2/1
  Sum4/1 -> R4/1

== system PC_drone_Simulation/SAV Control Mixing/+ Config Control Mixing 2 ==
  note: mc5 = + Psi _cor + Alt_cor
  note: + (plus) Drone Configuration Control Mixing
  note: mc6 = - Psi _cor + Alt_cor
  Psi Correction : Inport
  Alt Correction : Inport  Port=2
  Sum1 : Sum  Inputs=|++
  Sum3 : Sum  Inputs=+-|
  R5 : Outport
  R6 : Outport  Port=2
  wires:
  Sum3/1 -> R6/1
  Sum1/1 -> R5/1
  Psi Correction/1 -> Sum3/2, Sum1/1
  Alt Correction/1 -> Sum3/1, Sum1/2

== system PC_drone_Simulation/SAV Dynamics/External Disturbances ==
  note: Note: Torques are in units of N*m, Forces in N
      | Torques are applied to the BODY coordinate system.
      | Forces are applied from the WORLD coordinate system!
      | This can be changed by adjusting the equations within the S-function.
  Bus Creator : BusCreator  Inputs=6
  Bus to Vector : BusToVector
  Constant{2..6} (5 alike) : Constant  Value=0
  Step : Step  After=0  SampleTime=0
  "Disturbances " : Outport
  wires:
  Constant5/1 -> Bus Creator/6  "Force_z-axis"
  Constant4/1 -> Bus Creator/5  "Force_y-axis"
  Constant3/1 -> Bus Creator/4  "Force_x-axis"
  Constant2/1 -> Bus Creator/3  "Tau_bz-axis"
  Step/1 -> Bus Creator/2  "Tau_by-axis"
  Constant6/1 -> Bus Creator/1  "Tau_bx-axis"
  Bus Creator/1 -> Bus to Vector/1
  Bus to Vector/1 -> "Disturbances "/1

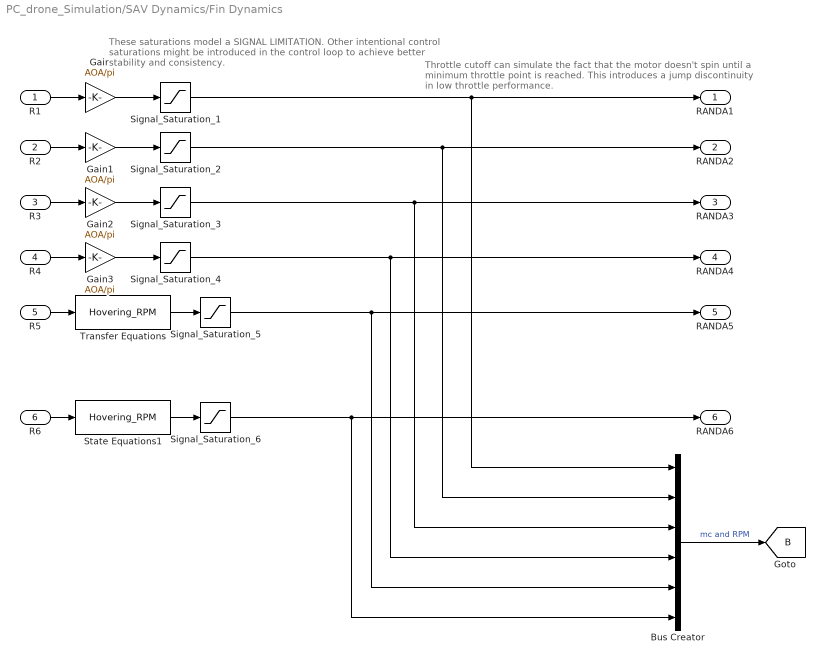
== system PC_drone_Simulation/SAV Dynamics/Fin Dynamics ==
  note: These saturations model a SIGNAL LIMITATION.
      | Other intentional control saturations might be introduced in the
      | control loop to achieve better stability and consistency.
  note: Throttle cutoff can simulate the fact that the motor doesn't
      | spin until a minimum throttle point is reached. This introduces
      | a jump discontinuity in low throttle performance.
  R1 : Inport
  R2 : Inport  Port=2
  R3 : Inport  Port=3
  R4 : Inport  Port=4
  R5 : Inport  Port=5
  R6 : Inport  Port=6
  Bus Creator : BusCreator  Inputs=6
  Gain{,1..3} (4 alike) : Gain  Gain=AOA/pi
  Signal_Saturation_{1..4} (4 alike) : Saturate  UpperLimit=AOA  LowerLimit=-AOA
  Signal_Saturation_5 : Saturate  UpperLimit=100  LowerLimit=50
  Signal_Saturation_6 : Saturate  UpperLimit=100  LowerLimit=50
  State Equations1 : M-S-Function  FunctionName=Hovering_RPM  Parameters=droneModel
      mask Display:
      | port_label('input', 1, 'Throttle2')
      | port_label('output', 1, 'RANDA6')
  Transfer Equations : M-S-Function  FunctionName=Hovering_RPM  Parameters=droneModel
      mask Display:
      | port_label('input', 1, 'Throttle1')
      | port_label('output', 1, 'RANDA5')
  RANDA1 : Outport
  RANDA2 : Outport  Port=2
  RANDA3 : Outport  Port=3
  RANDA4 : Outport  Port=4
  RANDA5 : Outport  Port=5
  RANDA6 : Outport  Port=6
  tag scope: B=global
  wires:
  Bus Creator/1 -> [B]  "mc and RPM"
  Signal_Saturation_4/1 -> RANDA4/1, Bus Creator/4
  Signal_Saturation_3/1 -> RANDA3/1, Bus Creator/3
  Signal_Saturation_2/1 -> RANDA2/1, Bus Creator/2
  Signal_Saturation_1/1 -> RANDA1/1, Bus Creator/1
  R3/1 -> Gain2/1
  R2/1 -> Gain1/1
  R4/1 -> Gain3/1
  R1/1 -> Gain/1
  Gain/1 -> Signal_Saturation_1/1
  Gain1/1 -> Signal_Saturation_2/1
  Gain2/1 -> Signal_Saturation_3/1
  Gain3/1 -> Signal_Saturation_4/1
  Signal_Saturation_5/1 -> RANDA5/1, Bus Creator/5
  Signal_Saturation_6/1 -> Bus Creator/6, RANDA6/1
  Transfer Equations/1 -> Signal_Saturation_5/1
  R5/1 -> Transfer Equations/1
  R6/1 -> State Equations1/1
  State Equations1/1 -> Signal_Saturation_6/1

== matlab function PC_drone_Simulation/Position Controller/Azimuth Command Control/MATLAB Function ==
  data: Vbx_error input; Vbazi_error output; Vbx input; Vby_error input; Vby input; Vbazi output
function [Vbazi_error,Vbazi] = CtoS(Vbx_error,Vbx,Vby_error,Vby)

% [Vbazi_error,junk1, junk2] = cart2sph(Vbx_error,Vby_error,0);
% [Vbazi,junk1,junk2] = cart2sph(Vbx,Vby,0);

Vbazi_error = atan2(Vby_error,Vbx_error);
Vbazi = atan2(Vby,Vbx);
